simulink model "dsa2k_iwave_rfi"  (R2021a)
settings: Solver=VariableStepAuto  StartTime=0.0  StopTime=10.0  RelTol=1e-3
undefined symbols (not defined in the file): datetime, i, posixtime
libraries: xbsIndex_r4 x3053, casper_library_misc x61, rtr_casper_dsp_lib x31, xps_library x1
(part 5 of 43)

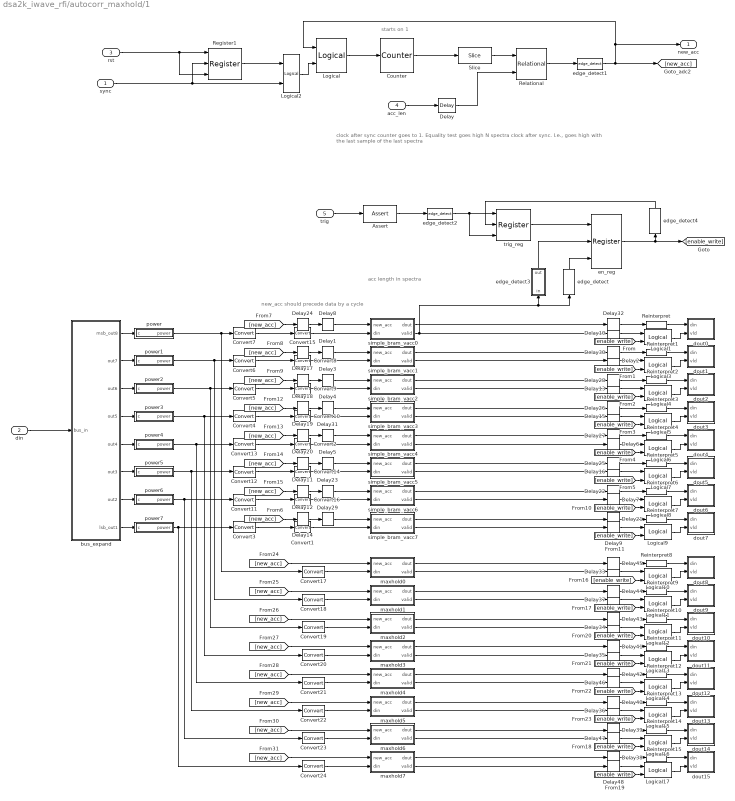
== system dsa2k_iwave_rfi/autocorr_maxhold/1 ==
  note: new_acc should precede data by a cycle
  note: acc length in spectra
  note: clock after sync counter goes to 1.
      |
      | Equality test goes high N spectra clock after sync. I.e., goes high with the last sample of the last spectra
  note: starts on 1
  sync : Inport
  din : Inport  Port=2
  rst : Inport  Port=3
  acc_len : Inport  Port=4
  trig : Inport  Port=5
  Assert : xbsIndex_r4/Assert  assert_type=off  type_source=Explicitly  gui_display_data_type=Fixed-point  arith_type="Signed  (2's comp)"  n_bits=16  bin_pt=14  preci_type=Single  exp_width=8  frac_width=24  assert_rate=on  rate_source=Explicitly  period=1  output_port=on  block_type=assert
  Convert{1..2,8..10,14..16} (8 alike) : xbsIndex_r4/Convert  gui_display_data_type=Floating-point  arith_type=Floating-point  n_bits=31  bin_pt=28  float_type=Single  exp_bits=8  fraction_bits=24  quantization="Round  (unbiased: Even Values)"  overflow=Wrap  en=off  latency=3  pipeline=on  dbl_ovrd=off  block_type=convert
  Convert{3..7,11..13} (8 alike) : xbsIndex_r4/Convert  gui_display_data_type=Fixed-point  arith_type="Signed  (2's comp)"  n_bits=37  bin_pt=34  float_type=Single  exp_bits=8  fraction_bits=24  quantization=Truncate  overflow=Wrap  en=off  latency=0  pipeline=off  dbl_ovrd=off  block_type=convert
  Convert{17..24} (8 alike) : xbsIndex_r4/Convert  gui_display_data_type=Fixed-point  arith_type=Unsigned  n_bits=32  bin_pt=30  float_type=Single  exp_bits=8  fraction_bits=24  quantization=Truncate  overflow=Wrap  en=off  latency=0  pipeline=off  dbl_ovrd=off  block_type=convert
  Counter : xbsIndex_r4/Counter  cnt_type=Free Running  cnt_to=Inf  operation=Up  start_count=1  cnt_by_val=1  arith_type=Unsigned  n_bits=30  bin_pt=0  load_pin=off  rst=on  en=off  explicit_period=on  period=1  use_behavioral_HDL=off  implementation=Fabric  dbl_ovrd=off  block_type=counter
  Delay{,2,6..7,9..10,13,15..16,33..37,46..48} (17 alike) : xbsIndex_r4/Delay  rst=off  infoeditControl=Selection of Reset will increase slice count due to use of real FFs and instead of SRLs  en=off  latency=1  reg_retiming=off  dbl_ovrd=off  block_type=delay
  Delay{1,3..5,8,23,29,31} (8 alike) : xbsIndex_r4/Delay  rst=off  infoeditControl=Selection of Reset will increase slice count due to use of real FFs and instead of SRLs  en=off  latency=4  reg_retiming=on  dbl_ovrd=off  block_type=delay
  Delay{11..12,14,17..20,24} (8 alike) : xbsIndex_r4/Delay  rst=off  infoeditControl=Selection of Reset will increase slice count due to use of real FFs and instead of SRLs  en=off  latency=3  reg_retiming=on  dbl_ovrd=off  block_type=delay
  Delay{21..22,25..28,30,32,38..45} (16 alike) : xbsIndex_r4/Delay  rst=off  infoeditControl=Selection of Reset will increase slice count due to use of real FFs and instead of SRLs  en=off  latency=1  reg_retiming=on  dbl_ovrd=off  block_type=delay
  Logical : xbsIndex_r4/Logical  logical_function=OR  inputs=2  en=off  latency=0  precision=Full  arith_type=Unsigned  n_bits=16  bin_pt=0  align_bp=on  dbl_ovrd=off  block_type=logical
  Logical{1..17} (17 alike) : xbsIndex_r4/Logical  logical_function=AND  inputs=2  en=off  latency=0  precision=Full  arith_type=Unsigned  n_bits=16  bin_pt=0  align_bp=on  dbl_ovrd=off  block_type=logical
  Register1 : xbsIndex_r4/Register  init=0  rst=on  en=on  dbl_ovrd=off  block_type=register
  Reinterpret{,1..15} (16 alike) : xbsIndex_r4/Reinterpret  force_arith_type=on  arith_type=Unsigned  force_bin_pt=on  bin_pt=0  block_type=reinterpret
  Relational : xbsIndex_r4/Relational  mode=a=b  op_type=Bool  en=off  latency=0  dbl_ovrd=off  block_type=relational
  Slice : xbsIndex_r4/Slice  nbits=30-nchan_bits-npol_bits  boolean_output=off  mode=Lower Bit Location + Width  bit1=0  base1=MSB of Input  bit0=nchan_bits + npol_bits  base0=LSB of Input  dbl_ovrd=off  block_type=slice
  bus_expand : Subsystem  AncestorBlock=casper_library_flow_control/bus_expand  mask(bus_expand){mode=divisions of equal size, outputNum=8, outputWidth=36, outputBinaryPt=0, outputArithmeticType=0, show_format=off, outputToWorkspace=off, variablePrefix=out, outputToModelAsWell=on}
      mask prompts: outputNum "Number of outputs:"; outputWidth "Output width:"; outputBinaryPt "Output binary point position:"; outputArithmeticType "Output arithmetic type (ufix=0, fix=1, bool=2):"; show_format "Print format string?"; outputToWorkspace "Output to workspace?"; variablePrefix "Variable name prefix:"; outputToModelAsWell "Output to model as well?"
      mask help:
      | Expands a 'bus' made using a bus_create or Xilinx
      | concat block.
      | The input will be divided into the specified number
      | of outputs with the specified arithmetic types.
      | Divisions are made from most significant bit.
      mask init: same as dsa2k_iwave_rfi/autocorr_maxhold/bus_expand
      settings: AttributesFormatString=8 outputs
      mask TypeOptions mode: divisions of equal size | divisions of arbitrary size
      mask Callback mode: %bus_expand_callback();
      mask Callback outputWidth: %bus_expand_callback();
      mask Callback outputToWorkspace: %bus_expand_callback();
  dout0 : Subsystem
  dout1 : Subsystem
  dout10 : Subsystem
  dout11 : Subsystem
  dout12 : Subsystem
  dout13 : Subsystem
  dout14 : Subsystem
  dout15 : Subsystem
  dout2 : Subsystem
  dout3 : Subsystem
  dout4 : Subsystem
  dout5 : Subsystem
  dout6 : Subsystem
  dout7 : Subsystem
  dout8 : Subsystem
  dout9 : Subsystem
  edge_detect{,1..2,4} (4 alike) : casper_library_misc/edge_detect  edge=Rising  polarity=Active High  x_in=[0 0.08 0.08 0.16 0.16 0.24 0.24 0.32 0.32 0.4]  y_in="[-1 -1  1  1  1  1  1  1  1  1]"  x_out=[0.6 0.68 0.68 0.76 0.76 0.84 0.84 0.92 0.92 1]  y_out="[-1 -1  1  1 -1 -1 -1 -1 -1 -1]"
  edge_detect3 : Subsystem  AncestorBlock=casper_library_misc/edge_detect  mask(edge_detect){edge=Falling, polarity=Active High, x_in=[0 0.08 0.08 0.16 0.16 0.24 0.24 0.32 0.32 0.4], y_in=[-1 -1  1  1  1  1  1  1  1  1], x_out=[0.6 0.68 0.68 0.76 0.76 0.84 0.84 0.92 0.92 1], y_out=[-1 -1  1  1 -1 -1 -1 -1 -1 -1]}
      mask prompts: edge "Edge Type"; polarity "Output Polarity"; x_in "Input X Positions"; y_in "Input Y Positions"; x_out "Output X Positions"; y_out "Output Y Positions"
      mask help: Output is active for one-cycle after each edge of the specified type (i.e. rising, falling or both).
      mask init: same as dsa2k_iwave_rfi/sync/ed1
      settings: AttributesFormatString=|
      | falling edges
      | active high
      mask Help: Output is active for one-cycle after each edge of the specified type (i.e. rising, falling, or both).  Latency is zero.
      mask TypeOptions edge: Rising | Falling | Both
      mask TypeOptions polarity: Active High | Active Low
      mask Display:
      | plot(x_in_num,0.5+y_in_num*0.2);
      | plot(x_out_num,0.5+y_out_num*0.2);
  en_reg : xbsIndex_r4/Register  init=0  rst=on  en=on  dbl_ovrd=off  block_type=register
  maxhold0 : Subsystem  AncestorBlock=casper_library_accumulators/simple_bram_vacc  mask(simple_bram_vacc){vec_len=2^(nchan_bits + npol_bits), arith_type=Unsigned, n_bits=32, bin_pt=30}
      mask prompts: vec_len "Vector length:"; arith_type "Output type:"; n_bits "Bit width (output):"; bin_pt "Binary point (output):"
      mask help: This simple vector accumulator is based on a shift register. It outputs its previous accumulated vector after a new_acc pulse is received.
      mask init:
      | % simple_bram_vacc_init(gcb, ...
      | %     'vec_len', vec_len, ...
      | %     'arith_type', arith_type, ...
      | %     'n_bits', n_bits, ...
      | %     'bin_pt', bin_pt);
      mask TypeOptions arith_type: Signed | Unsigned
  maxhold1 : Subsystem  AncestorBlock=casper_library_accumulators/simple_bram_vacc  mask(simple_bram_vacc){vec_len=2^(nchan_bits + npol_bits), arith_type=Unsigned, n_bits=32, bin_pt=30}
      mask prompts: vec_len "Vector length:"; arith_type "Output type:"; n_bits "Bit width (output):"; bin_pt "Binary point (output):"
      mask help: This simple vector accumulator is based on a shift register. It outputs its previous accumulated vector after a new_acc pulse is received.
      mask init:
      | % simple_bram_vacc_init(gcb, ...
      | %     'vec_len', vec_len, ...
      | %     'arith_type', arith_type, ...
      | %     'n_bits', n_bits, ...
      | %     'bin_pt', bin_pt);
      mask TypeOptions arith_type: Signed | Unsigned
  maxhold2 : Subsystem  AncestorBlock=casper_library_accumulators/simple_bram_vacc  mask(simple_bram_vacc){vec_len=2^(nchan_bits + npol_bits), arith_type=Unsigned, n_bits=32, bin_pt=30}
      mask prompts: vec_len "Vector length:"; arith_type "Output type:"; n_bits "Bit width (output):"; bin_pt "Binary point (output):"
      mask help: This simple vector accumulator is based on a shift register. It outputs its previous accumulated vector after a new_acc pulse is received.
      mask init:
      | % simple_bram_vacc_init(gcb, ...
      | %     'vec_len', vec_len, ...
      | %     'arith_type', arith_type, ...
      | %     'n_bits', n_bits, ...
      | %     'bin_pt', bin_pt);
      mask TypeOptions arith_type: Signed | Unsigned
  maxhold3 : Subsystem  AncestorBlock=casper_library_accumulators/simple_bram_vacc  mask(simple_bram_vacc){vec_len=2^(nchan_bits + npol_bits), arith_type=Unsigned, n_bits=32, bin_pt=30}
      mask prompts: vec_len "Vector length:"; arith_type "Output type:"; n_bits "Bit width (output):"; bin_pt "Binary point (output):"
      mask help: This simple vector accumulator is based on a shift register. It outputs its previous accumulated vector after a new_acc pulse is received.
      mask init:
      | % simple_bram_vacc_init(gcb, ...
      | %     'vec_len', vec_len, ...
      | %     'arith_type', arith_type, ...
      | %     'n_bits', n_bits, ...
      | %     'bin_pt', bin_pt);
      mask TypeOptions arith_type: Signed | Unsigned
  maxhold4 : Subsystem  AncestorBlock=casper_library_accumulators/simple_bram_vacc  mask(simple_bram_vacc){vec_len=2^(nchan_bits + npol_bits), arith_type=Unsigned, n_bits=32, bin_pt=30}
      mask prompts: vec_len "Vector length:"; arith_type "Output type:"; n_bits "Bit width (output):"; bin_pt "Binary point (output):"
      mask help: This simple vector accumulator is based on a shift register. It outputs its previous accumulated vector after a new_acc pulse is received.
      mask init:
      | % simple_bram_vacc_init(gcb, ...
      | %     'vec_len', vec_len, ...
      | %     'arith_type', arith_type, ...
      | %     'n_bits', n_bits, ...
      | %     'bin_pt', bin_pt);
      mask TypeOptions arith_type: Signed | Unsigned
  maxhold5 : Subsystem  AncestorBlock=casper_library_accumulators/simple_bram_vacc  mask(simple_bram_vacc){vec_len=2^(nchan_bits + npol_bits), arith_type=Unsigned, n_bits=32, bin_pt=30}
      mask prompts: vec_len "Vector length:"; arith_type "Output type:"; n_bits "Bit width (output):"; bin_pt "Binary point (output):"
      mask help: This simple vector accumulator is based on a shift register. It outputs its previous accumulated vector after a new_acc pulse is received.
      mask init:
      | % simple_bram_vacc_init(gcb, ...
      | %     'vec_len', vec_len, ...
      | %     'arith_type', arith_type, ...
      | %     'n_bits', n_bits, ...
      | %     'bin_pt', bin_pt);
      mask TypeOptions arith_type: Signed | Unsigned
  maxhold6 : Subsystem  AncestorBlock=casper_library_accumulators/simple_bram_vacc  mask(simple_bram_vacc){vec_len=2^(nchan_bits + npol_bits), arith_type=Unsigned, n_bits=32, bin_pt=30}
      mask prompts: vec_len "Vector length:"; arith_type "Output type:"; n_bits "Bit width (output):"; bin_pt "Binary point (output):"
      mask help: This simple vector accumulator is based on a shift register. It outputs its previous accumulated vector after a new_acc pulse is received.
      mask init:
      | % simple_bram_vacc_init(gcb, ...
      | %     'vec_len', vec_len, ...
      | %     'arith_type', arith_type, ...
      | %     'n_bits', n_bits, ...
      | %     'bin_pt', bin_pt);
      mask TypeOptions arith_type: Signed | Unsigned
  maxhold7 : Subsystem  AncestorBlock=casper_library_accumulators/simple_bram_vacc  mask(simple_bram_vacc){vec_len=2^(nchan_bits + npol_bits), arith_type=Unsigned, n_bits=32, bin_pt=30}
      mask prompts: vec_len "Vector length:"; arith_type "Output type:"; n_bits "Bit width (output):"; bin_pt "Binary point (output):"
      mask help: This simple vector accumulator is based on a shift register. It outputs its previous accumulated vector after a new_acc pulse is received.
      mask init:
      | % simple_bram_vacc_init(gcb, ...
      | %     'vec_len', vec_len, ...
      | %     'arith_type', arith_type, ...
      | %     'n_bits', n_bits, ...
      | %     'bin_pt', bin_pt);
      mask TypeOptions arith_type: Signed | Unsigned
  power : Subsystem  mask(power){BitWidth=18, add_latency=1, mult_latency=3}
      mask prompts: BitWidth "Bit Width"; add_latency "Add Latency"; mult_latency "Mult Latency"
      mask help: Squares real and imaginary components of complex input and adds them.
      mask Help: eval('xlWeb(''http://casper.berkeley.edu/wiki/Power'')')
      mask Display:
      | port_label('input', 1, 'c');
      | port_label('output', 1, 'power');
      | disp(['Z^-', num2str(mult_latency+add_latency)]);
  power1 : Subsystem  mask(power){BitWidth=18, add_latency=1, mult_latency=3}
      mask prompts: BitWidth "Bit Width"; add_latency "Add Latency"; mult_latency "Mult Latency"
      mask help: Squares real and imaginary components of complex input and adds them.
      mask Help: eval('xlWeb(''http://casper.berkeley.edu/wiki/Power'')')
      mask Display:
      | port_label('input', 1, 'c');
      | port_label('output', 1, 'power');
      | disp(['Z^-', num2str(mult_latency+add_latency)]);
  power2 : Subsystem  mask(power){BitWidth=18, add_latency=1, mult_latency=3}
      mask prompts: BitWidth "Bit Width"; add_latency "Add Latency"; mult_latency "Mult Latency"
      mask help: Squares real and imaginary components of complex input and adds them.
      mask Help: eval('xlWeb(''http://casper.berkeley.edu/wiki/Power'')')
      mask Display:
      | port_label('input', 1, 'c');
      | port_label('output', 1, 'power');
      | disp(['Z^-', num2str(mult_latency+add_latency)]);
  power3 : Subsystem  mask(power){BitWidth=18, add_latency=1, mult_latency=3}
      mask prompts: BitWidth "Bit Width"; add_latency "Add Latency"; mult_latency "Mult Latency"
      mask help: Squares real and imaginary components of complex input and adds them.
      mask Help: eval('xlWeb(''http://casper.berkeley.edu/wiki/Power'')')
      mask Display:
      | port_label('input', 1, 'c');
      | port_label('output', 1, 'power');
      | disp(['Z^-', num2str(mult_latency+add_latency)]);
  power4 : Subsystem  mask(power){BitWidth=18, add_latency=1, mult_latency=3}
      mask prompts: BitWidth "Bit Width"; add_latency "Add Latency"; mult_latency "Mult Latency"
      mask help: Squares real and imaginary components of complex input and adds them.
      mask Help: eval('xlWeb(''http://casper.berkeley.edu/wiki/Power'')')
      mask Display:
      | port_label('input', 1, 'c');
      | port_label('output', 1, 'power');
      | disp(['Z^-', num2str(mult_latency+add_latency)]);
  power5 : Subsystem  mask(power){BitWidth=18, add_latency=1, mult_latency=3}
      mask prompts: BitWidth "Bit Width"; add_latency "Add Latency"; mult_latency "Mult Latency"
      mask help: Squares real and imaginary components of complex input and adds them.
      mask Help: eval('xlWeb(''http://casper.berkeley.edu/wiki/Power'')')
      mask Display:
      | port_label('input', 1, 'c');
      | port_label('output', 1, 'power');
      | disp(['Z^-', num2str(mult_latency+add_latency)]);
  power6 : Subsystem  mask(power){BitWidth=18, add_latency=1, mult_latency=3}
      mask prompts: BitWidth "Bit Width"; add_latency "Add Latency"; mult_latency "Mult Latency"
      mask help: Squares real and imaginary components of complex input and adds them.
      mask Help: eval('xlWeb(''http://casper.berkeley.edu/wiki/Power'')')
      mask Display:
      | port_label('input', 1, 'c');
      | port_label('output', 1, 'power');
      | disp(['Z^-', num2str(mult_latency+add_latency)]);
  power7 : Subsystem  mask(power){BitWidth=18, add_latency=1, mult_latency=3}
      mask prompts: BitWidth "Bit Width"; add_latency "Add Latency"; mult_latency "Mult Latency"
      mask help: Squares real and imaginary components of complex input and adds them.
      mask Help: eval('xlWeb(''http://casper.berkeley.edu/wiki/Power'')')
      mask Display:
      | port_label('input', 1, 'c');
      | port_label('output', 1, 'power');
      | disp(['Z^-', num2str(mult_latency+add_latency)]);
  simple_bram_vacc0 : Subsystem  AncestorBlock=casper_library_accumulators/simple_bram_vacc  mask(simple_bram_vacc){vec_len=2^(nchan_bits + npol_bits), arith_type=Signed, n_bits=30 + 17, bin_pt=28}
      mask prompts: vec_len "Vector length:"; arith_type "Output type:"; n_bits "Bit width (output):"; bin_pt "Binary point (output):"
      mask help: This simple vector accumulator is based on a shift register. It outputs its previous accumulated vector after a new_acc pulse is received.
      mask init:
      | simple_bram_vacc_init(gcb, ...
      |     'vec_len', vec_len, ...
      |     'arith_type', arith_type, ...
      |     'n_bits', n_bits, ...
      |     'bin_pt', bin_pt);
      mask TypeOptions arith_type: Signed | Unsigned
  simple_bram_vacc1 : Subsystem  AncestorBlock=casper_library_accumulators/simple_bram_vacc  mask(simple_bram_vacc){vec_len=2^(nchan_bits + npol_bits), arith_type=Signed, n_bits=30 + 17, bin_pt=28}
      mask prompts: vec_len "Vector length:"; arith_type "Output type:"; n_bits "Bit width (output):"; bin_pt "Binary point (output):"
      mask help: This simple vector accumulator is based on a shift register. It outputs its previous accumulated vector after a new_acc pulse is received.
      mask init:
      | simple_bram_vacc_init(gcb, ...
      |     'vec_len', vec_len, ...
      |     'arith_type', arith_type, ...
      |     'n_bits', n_bits, ...
      |     'bin_pt', bin_pt);
      mask TypeOptions arith_type: Signed | Unsigned
  simple_bram_vacc2 : Subsystem  AncestorBlock=casper_library_accumulators/simple_bram_vacc  mask(simple_bram_vacc){vec_len=2^(nchan_bits + npol_bits), arith_type=Signed, n_bits=30 + 17, bin_pt=28}
      mask prompts: vec_len "Vector length:"; arith_type "Output type:"; n_bits "Bit width (output):"; bin_pt "Binary point (output):"
      mask help: This simple vector accumulator is based on a shift register. It outputs its previous accumulated vector after a new_acc pulse is received.
      mask init:
      | simple_bram_vacc_init(gcb, ...
      |     'vec_len', vec_len, ...
      |     'arith_type', arith_type, ...
      |     'n_bits', n_bits, ...
      |     'bin_pt', bin_pt);
      mask TypeOptions arith_type: Signed | Unsigned
  simple_bram_vacc3 : Subsystem  AncestorBlock=casper_library_accumulators/simple_bram_vacc  mask(simple_bram_vacc){vec_len=2^(nchan_bits + npol_bits), arith_type=Signed, n_bits=30 + 17, bin_pt=28}
      mask prompts: vec_len "Vector length:"; arith_type "Output type:"; n_bits "Bit width (output):"; bin_pt "Binary point (output):"
      mask help: This simple vector accumulator is based on a shift register. It outputs its previous accumulated vector after a new_acc pulse is received.
      mask init:
      | simple_bram_vacc_init(gcb, ...
      |     'vec_len', vec_len, ...
      |     'arith_type', arith_type, ...
      |     'n_bits', n_bits, ...
      |     'bin_pt', bin_pt);
      mask TypeOptions arith_type: Signed | Unsigned
  simple_bram_vacc4 : Subsystem  AncestorBlock=casper_library_accumulators/simple_bram_vacc  mask(simple_bram_vacc){vec_len=2^(nchan_bits + npol_bits), arith_type=Signed, n_bits=30 + 17, bin_pt=28}
      mask prompts: vec_len "Vector length:"; arith_type "Output type:"; n_bits "Bit width (output):"; bin_pt "Binary point (output):"
      mask help: This simple vector accumulator is based on a shift register. It outputs its previous accumulated vector after a new_acc pulse is received.
      mask init:
      | simple_bram_vacc_init(gcb, ...
      |     'vec_len', vec_len, ...
      |     'arith_type', arith_type, ...
      |     'n_bits', n_bits, ...
      |     'bin_pt', bin_pt);
      mask TypeOptions arith_type: Signed | Unsigned
  simple_bram_vacc5 : Subsystem  AncestorBlock=casper_library_accumulators/simple_bram_vacc  mask(simple_bram_vacc){vec_len=2^(nchan_bits + npol_bits), arith_type=Signed, n_bits=30 + 17, bin_pt=28}
      mask prompts: vec_len "Vector length:"; arith_type "Output type:"; n_bits "Bit width (output):"; bin_pt "Binary point (output):"
      mask help: This simple vector accumulator is based on a shift register. It outputs its previous accumulated vector after a new_acc pulse is received.
      mask init:
      | simple_bram_vacc_init(gcb, ...
      |     'vec_len', vec_len, ...
      |     'arith_type', arith_type, ...
      |     'n_bits', n_bits, ...
      |     'bin_pt', bin_pt);
      mask TypeOptions arith_type: Signed | Unsigned
  simple_bram_vacc6 : Subsystem  AncestorBlock=casper_library_accumulators/simple_bram_vacc  mask(simple_bram_vacc){vec_len=2^(nchan_bits + npol_bits), arith_type=Signed, n_bits=30 + 17, bin_pt=28}
      mask prompts: vec_len "Vector length:"; arith_type "Output type:"; n_bits "Bit width (output):"; bin_pt "Binary point (output):"
      mask help: This simple vector accumulator is based on a shift register. It outputs its previous accumulated vector after a new_acc pulse is received.
      mask init:
      | simple_bram_vacc_init(gcb, ...
      |     'vec_len', vec_len, ...
      |     'arith_type', arith_type, ...
      |     'n_bits', n_bits, ...
      |     'bin_pt', bin_pt);
      mask TypeOptions arith_type: Signed | Unsigned
  simple_bram_vacc7 : Subsystem  AncestorBlock=casper_library_accumulators/simple_bram_vacc  mask(simple_bram_vacc){vec_len=2^(nchan_bits + npol_bits), arith_type=Signed, n_bits=30 + 17, bin_pt=28}
      mask prompts: vec_len "Vector length:"; arith_type "Output type:"; n_bits "Bit width (output):"; bin_pt "Binary point (output):"
      mask help: This simple vector accumulator is based on a shift register. It outputs its previous accumulated vector after a new_acc pulse is received.
      mask init:
      | simple_bram_vacc_init(gcb, ...
      |     'vec_len', vec_len, ...
      |     'arith_type', arith_type, ...
      |     'n_bits', n_bits, ...
      |     'bin_pt', bin_pt);
      mask TypeOptions arith_type: Signed | Unsigned
  trig_reg : xbsIndex_r4/Register  init=0  rst=on  en=on  dbl_ovrd=off  block_type=register
  new_acc : Outport  VectorParamsAs1DForOutWhenUnconnected=off
  wires:
  Delay31/1 -> simple_bram_vacc4/1(new_acc)
  Delay5/1 -> simple_bram_vacc5/1(new_acc)
  Delay23/1 -> simple_bram_vacc6/1(new_acc)
  Delay29/1 -> simple_bram_vacc7/1(new_acc)
  power7/1(power) -> Convert3/1, Convert24/1
  power6/1(power) -> Convert11/1, Convert23/1
  power5/1(power) -> Convert12/1, Convert22/1
  power4/1(power) -> Convert13/1, Convert21/1
  [new_acc] -> Delay14/1
  [new_acc] -> Delay12/1
  [new_acc] -> Delay11/1
  [new_acc] -> Delay20/1
  Logical6/1 -> dout4/2(vld)
  [enable_write] -> Logical6/2
  [enable_write] -> Logical7/2
  Logical7/1 -> dout5/2(vld)
  Logical8/1 -> dout6/2(vld)
  [enable_write] -> Logical8/2
  [enable_write] -> Logical9/2
  Logical9/1 -> dout7/2(vld)
  simple_bram_vacc4/1(dout) -> Delay27/1
  simple_bram_vacc5/1(dout) -> Delay25/1
  simple_bram_vacc6/1(dout) -> Delay22/1
  simple_bram_vacc6/2(valid) -> Delay7/1
  simple_bram_vacc7/1(dout) -> Delay21/1
  simple_bram_vacc7/2(valid) -> Delay9/1
  simple_bram_vacc5/2(valid) -> Delay16/1
  simple_bram_vacc4/2(valid) -> Delay6/1
  Delay14/1 -> Delay29/1
  Convert1/1 -> simple_bram_vacc7/2(din)
  Delay12/1 -> Delay23/1
  Convert16/1 -> simple_bram_vacc6/2(din)
  Convert14/1 -> simple_bram_vacc5/2(din)
  Delay11/1 -> Delay5/1
  Delay20/1 -> Delay31/1
  Convert2/1 -> simple_bram_vacc4/2(din)
  Delay27/1 -> Reinterpret4/1
  Delay6/1 -> Logical6/1
  Delay25/1 -> Reinterpret5/1
  Delay16/1 -> Logical7/1
  Delay22/1 -> Reinterpret6/1
  Delay7/1 -> Logical8/1
  Delay9/1 -> Logical9/1
  Delay21/1 -> Reinterpret7/1
  Convert3/1 -> Convert1/1
  Convert11/1 -> Convert16/1
  Convert12/1 -> Convert14/1
  Convert13/1 -> Convert2/1
  Reinterpret4/1 -> dout4/1(din)
  Reinterpret5/1 -> dout5/1(din)
  Reinterpret6/1 -> dout6/1(din)
  Reinterpret7/1 -> dout7/1(din)
  Reinterpret3/1 -> dout3/1(din)
  Reinterpret2/1 -> dout2/1(din)
  Reinterpret1/1 -> dout1/1(din)
  Reinterpret/1 -> dout0/1(din)
  Convert7/1 -> Convert15/1
  Convert6/1 -> Convert8/1
  Convert5/1 -> Convert9/1
  Convert4/1 -> Convert10/1
  Delay26/1 -> Reinterpret3/1
  Delay15/1 -> Logical5/1
  Delay13/1 -> Logical4/1
  Delay28/1 -> Reinterpret2/1
  Delay2/1 -> Logical3/1
  Delay30/1 -> Reinterpret1/1
  Delay10/1 -> Logical1/1
  Delay32/1 -> Reinterpret/1
  Convert15/1 -> simple_bram_vacc0/2(din)
  Delay24/1 -> Delay8/1
  Delay17/1 -> Delay1/1
  Convert8/1 -> simple_bram_vacc1/2(din)
  Convert9/1 -> simple_bram_vacc2/2(din)
  Delay18/1 -> Delay3/1
  Convert10/1 -> simple_bram_vacc3/2(din)
  Delay19/1 -> Delay4/1
  simple_bram_vacc0/2(valid) -> edge_detect3/1(in), edge_detect/1, Delay10/1
  simple_bram_vacc1/2(valid) -> Delay2/1
  simple_bram_vacc3/2(valid) -> Delay15/1
  simple_bram_vacc3/1(dout) -> Delay26/1
  simple_bram_vacc2/2(valid) -> Delay13/1
  simple_bram_vacc2/1(dout) -> Delay28/1
  simple_bram_vacc1/1(dout) -> Delay30/1
  simple_bram_vacc0/1(dout) -> Delay32/1
  Assert/1 -> edge_detect2/1
  trig/1 -> Assert/1
  Logical5/1 -> dout3/2(vld)
  [enable_write] -> Logical5/2
  [enable_write] -> Logical4/2
  Logical4/1 -> dout2/2(vld)
  Logical3/1 -> dout1/2(vld)
  [enable_write] -> Logical3/2
  [enable_write] -> Logical1/2
  en_reg/1 -> edge_detect4/1, [enable_write]
  Logical1/1 -> dout0/2(vld)
  edge_detect4/1 -> trig_reg/2
  edge_detect3/1(out) -> en_reg/2
  edge_detect/1 -> en_reg/3
  edge_detect2/1 -> trig_reg/1, trig_reg/3
  trig_reg/1 -> en_reg/1
  sync/1 -> Register1/2, Logical2/2
  Register1/1 -> Logical2/1
  rst/1 -> Register1/3, Register1/1
  edge_detect1/1 -> Logical/1, new_acc/1, [new_acc]
  Logical/1 -> Counter/1
  Counter/1 -> Slice/1
  [new_acc] -> Delay24/1
  [new_acc] -> Delay17/1
  [new_acc] -> Delay18/1
  [new_acc] -> Delay19/1
  power/1(power) -> Convert17/1, Convert7/1
  power1/1(power) -> Convert6/1, Convert18/1
  power2/1(power) -> Convert5/1, Convert19/1
  power3/1(power) -> Convert4/1, Convert20/1
  din/1 -> bus_expand/1(bus_in)
  Slice/1 -> Relational/1
  Relational/1 -> edge_detect1/1
  Logical2/1 -> Logical/2
  acc_len/1 -> Delay/1
  Delay4/1 -> simple_bram_vacc3/1(new_acc)
  Delay3/1 -> simple_bram_vacc2/1(new_acc)
  Delay1/1 -> simple_bram_vacc1/1(new_acc)
  Delay8/1 -> simple_bram_vacc0/1(new_acc)
  Delay/1 -> Relational/2
  bus_expand/1(msb_out8) -> power/1(c)
  bus_expand/2(out7) -> power1/1(c)
  bus_expand/3(out6) -> power2/1(c)
  bus_expand/4(out5) -> power3/1(c)
  bus_expand/5(out4) -> power4/1(c)
  bus_expand/6(out3) -> power5/1(c)
  bus_expand/7(out2) -> power6/1(c)
  bus_expand/8(lsb_out1) -> power7/1(c)
  Logical10/1 -> dout8/2(vld)
  [enable_write] -> Logical10/2
  [enable_write] -> Logical11/2
  Logical11/1 -> dout9/2(vld)
  Logical12/1 -> dout10/2(vld)
  [enable_write] -> Logical12/2
  [enable_write] -> Logical13/2
  Logical13/1 -> dout11/2(vld)
  maxhold0/1(dout) -> Delay45/1
  maxhold1/1(dout) -> Delay44/1
  maxhold2/1(dout) -> Delay43/1
  maxhold2/2(valid) -> Delay34/1
  maxhold3/1(dout) -> Delay41/1
  maxhold3/2(valid) -> Delay35/1
  maxhold1/2(valid) -> Delay37/1
  maxhold0/2(valid) -> Delay33/1
  Delay45/1 -> Reinterpret8/1
  Delay33/1 -> Logical10/1
  Delay44/1 -> Reinterpret9/1
  Delay37/1 -> Logical11/1
  Delay43/1 -> Reinterpret10/1
  Delay34/1 -> Logical12/1
  Delay35/1 -> Logical13/1
  Delay41/1 -> Reinterpret11/1
  Reinterpret8/1 -> dout8/1(din)
  Reinterpret9/1 -> dout9/1(din)
  Reinterpret10/1 -> dout10/1(din)
  Reinterpret11/1 -> dout11/1(din)
  Reinterpret15/1 -> dout15/1(din)
  Reinterpret14/1 -> dout14/1(din)
  Reinterpret13/1 -> dout13/1(din)
  Reinterpret12/1 -> dout12/1(din)
  Delay38/1 -> Reinterpret15/1
  Delay48/1 -> Logical17/1
  Delay47/1 -> Logical16/1
  Delay39/1 -> Reinterpret14/1
  Delay36/1 -> Logical15/1
  Delay40/1 -> Reinterpret13/1
  Delay46/1 -> Logical14/1
  Delay42/1 -> Reinterpret12/1
  maxhold4/2(valid) -> Delay46/1
  maxhold5/2(valid) -> Delay36/1
  maxhold7/2(valid) -> Delay48/1
  maxhold7/1(dout) -> Delay38/1
  maxhold6/2(valid) -> Delay47/1
  maxhold6/1(dout) -> Delay39/1
  maxhold5/1(dout) -> Delay40/1
  maxhold4/1(dout) -> Delay42/1
  Logical17/1 -> dout15/2(vld)
  [enable_write] -> Logical17/2
  [enable_write] -> Logical16/2
  Logical16/1 -> dout14/2(vld)
  Logical15/1 -> dout13/2(vld)
  [enable_write] -> Logical15/2
  [enable_write] -> Logical14/2
  Logical14/1 -> dout12/2(vld)
  [new_acc] -> maxhold0/1(new_acc)
  Convert17/1 -> maxhold0/2(din)
  [new_acc] -> maxhold1/1(new_acc)
  Convert18/1 -> maxhold1/2(din)
  [new_acc] -> maxhold2/1(new_acc)
  Convert19/1 -> maxhold2/2(din)
  [new_acc] -> maxhold3/1(new_acc)
  Convert20/1 -> maxhold3/2(din)
  Convert21/1 -> maxhold4/2(din)
  [new_acc] -> maxhold4/1(new_acc)
  [new_acc] -> maxhold5/1(new_acc)
  Convert22/1 -> maxhold5/2(din)
  Convert23/1 -> maxhold6/2(din)
  [new_acc] -> maxhold6/1(new_acc)
  [new_acc] -> maxhold7/1(new_acc)
  Convert24/1 -> maxhold7/2(din)

== system dsa2k_iwave_rfi/autocorr_maxhold/acc_cnt ==
  out_reg : Inport
  assert_reg : xbsIndex_r4/Assert  assert_type=on  type_source=Explicitly  gui_display_data_type=Fixed-point  arith_type=Unsigned  n_bits=32  bin_pt=0  preci_type=Single  exp_width=8  frac_width=24  assert_rate=off  rate_source=Explicitly  period=1  output_port=on  block_type=assert
  cast_gw : xbsIndex_r4/Convert  gui_display_data_type=Fixed-point  arith_type=Unsigned  n_bits=32  bin_pt=0  float_type=Single  exp_bits=8  fraction_bits=24  quantization=Truncate  overflow=Wrap  en=off  latency=1  pipeline=off  dbl_ovrd=off  block_type=convert
  dsa2k_iwave_rfi_autocorr_maxhold_acc_cnt_user_data_in : xbsIndex_r4/Gateway Out  inherit_from_input=off  hdl_port=on  rows=1  columns=1  UseAsDAC=off  DACChannel='1'  interface=None  automatic_assignment=on  address_offset=hex2dec('00')  intf_name=''  intf_description=''  timing_constraint=None  locs_specified=off  LOCs={}  io_standard={}  block_type=gatewayout
  io_delay : xbsIndex_r4/Delay  rst=off  infoeditControl=Selection of Reset will increase slice count due to use of real FFs and instead of SRLs  en=off  latency=0  reg_retiming=on  dbl_ovrd=off  block_type=delay
  reint1 : xbsIndex_r4/Reinterpret  force_arith_type=on  arith_type=Unsigned  force_bin_pt=on  bin_pt=0  block_type=reinterpret
  sim_out : Terminator
  sim_out_reg_gw : xbsIndex_r4/Gateway Out  inherit_from_input=off  hdl_port=off  rows=1  columns=1  UseAsDAC=off  DACChannel='1'  interface=None  automatic_assignment=on  address_offset=hex2dec('00')  intf_name=''  intf_description=''  timing_constraint=None  locs_specified=off  LOCs={}  io_standard={}  block_type=gatewayout
  sim_out_reg_sim_delay : xbsIndex_r4/Delay  rst=off  infoeditControl=Selection of Reset will increase slice count due to use of real FFs and instead of SRLs  en=off  latency=1  reg_retiming=on  dbl_ovrd=off  block_type=delay
  sim_out_reg : Outport  VectorParamsAs1DForOutWhenUnconnected=off
  wires:
  sim_out_reg_sim_delay/1 -> sim_out_reg_gw/1
  sim_out_reg_gw/1 -> sim_out_reg/1
  io_delay/1 -> cast_gw/1
  cast_gw/1 -> dsa2k_iwave_rfi_autocorr_maxhold_acc_cnt_user_data_in/1
  dsa2k_iwave_rfi_autocorr_maxhold_acc_cnt_user_data_in/1 -> sim_out/1
  out_reg/1 -> sim_out_reg_sim_delay/1, assert_reg/1
  assert_reg/1 -> reint1/1
  reint1/1 -> io_delay/1

== system dsa2k_iwave_rfi/autocorr_maxhold/acc_len ==
  sim_1 : Inport
  convert1_1 : DataTypeConversion  OutDataTypeStr=fixdt('ufix32_En0')  LockScale=on
  convert2_1 : DataTypeConversion  OutDataTypeStr=fixdt('ufix32_En0')  ConvertRealWorld=Stored Integer (SI)  LockScale=on
  dsa2k_iwave_rfi_autocorr_maxhold_acc_len_user_data_out : xbsIndex_r4/Gateway In  gui_display_data_type=Fixed-point  arith_type=Unsigned  n_bits=32  bin_pt=0  preci_type=Single  exp_width=8  frac_width=24  rows=1  columns=1  quantization="Round  (unbiased: +/- Inf)"  overflow=Saturate  period=1  UseAsADC=off  ADCChannel='1'  interface=None  automatic_assignment=on  address_offset=hex2dec('00')  intf_name=''  intf_description=''  default_value=0  timing_constraint=None  locs_specified=off  LOCs={}  io_standard={}  inherit_from_input=off  hdl_port=on  dbl_ovrd=off  block_type=gatewayin
  gain_1 : Gain  OutDataTypeStr=fixdt('ufix32_En0')
  io_delay : xbsIndex_r4/Delay  rst=off  infoeditControl=Selection of Reset will increase slice count due to use of real FFs and instead of SRLs  en=off  latency=0  reg_retiming=on  dbl_ovrd=off  block_type=delay
  reint1 : xbsIndex_r4/Reinterpret  force_arith_type=on  arith_type=Unsigned  force_bin_pt=on  bin_pt=0  block_type=reinterpret
  slice_reg : xbsIndex_r4/Slice  nbits=32  boolean_output=off  mode=Lower Bit Location + Width  bit1=0  base1=MSB of Input  bit0=0  base0=LSB of Input  dbl_ovrd=off  block_type=slice
  in_reg : Outport  VectorParamsAs1DForOutWhenUnconnected=off
  wires:
  dsa2k_iwave_rfi_autocorr_maxhold_acc_len_user_data_out/1 -> io_delay/1
  sim_1/1 -> convert1_1/1
  convert1_1/1 -> convert2_1/1
  convert2_1/1 -> gain_1/1
  gain_1/1 -> dsa2k_iwave_rfi_autocorr_maxhold_acc_len_user_data_out/1
  io_delay/1 -> slice_reg/1
  slice_reg/1 -> reint1/1
  reint1/1 -> in_reg/1

== system dsa2k_iwave_rfi/autocorr_maxhold/block_info ==
  info : Subsystem  Tag=casper:info  mask(comment_block){info={"library":"rtr","block_type":"rtr:autocorr-maxhold","block_name":"dsa2k_iwave_rfi/autocorr_maxhold","rev_major":1,"rev_minor":0,"n_chan_serial_bits":11,"n_chan_parallel_bits":3,"n_input_serial_bits":0,"n_input":2}}
      mask help:
      | Any comment made using this block will be parsed by the toolflow and stored in the bitstream, accessible by software.
      | It's an unevaluated string, and some characters make Matlab unhappy, so the user must define/find a data transport format if that is the intended purpose.
      settings: MoveFcn=pos = get_param(gcb, 'Position'); height = pos(4)-pos(2); txt = get_param(gcb, 'info'); set_param(gcb,'MaskValueString',txt);
      mask Display:
      | pos = get_param(gcb, 'Position');
      | height = pos(4)-pos(2);
      | txt = get_param(gcb, 'info');
      | text(10,height/2,txt);

== system dsa2k_iwave_rfi/autocorr_maxhold/bus_expand ==
  bus_in : Inport
  reinterpret1 : xbsIndex_r4/Reinterpret  force_arith_type=on  arith_type=Unsigned  force_bin_pt=on  bin_pt=0  block_type=reinterpret
  reinterpret2 : xbsIndex_r4/Reinterpret  force_arith_type=on  arith_type=Unsigned  force_bin_pt=on  bin_pt=0  block_type=reinterpret
  slice1 : xbsIndex_r4/Slice  nbits=288  boolean_output=off  mode=Upper Bit Location + Width  bit1=-288  base1=MSB of Input  bit0=0  base0=LSB of Input  dbl_ovrd=off  block_type=slice
  slice2 : xbsIndex_r4/Slice  nbits=288  boolean_output=off  mode=Upper Bit Location + Width  bit1=0  base1=MSB of Input  bit0=0  base0=LSB of Input  dbl_ovrd=off  block_type=slice
  msb_out2 : Outport  VectorParamsAs1DForOutWhenUnconnected=off
  lsb_out1 : Outport  Port=2  VectorParamsAs1DForOutWhenUnconnected=off
  wires:
  bus_in/1 -> slice2/1, slice1/1
  slice2/1 -> reinterpret2/1
  reinterpret2/1 -> msb_out2/1
  slice1/1 -> reinterpret1/1
  reinterpret1/1 -> lsb_out1/1

== system dsa2k_iwave_rfi/autocorr_maxhold/trig ==
  sim_1 : Inport
  convert1_1 : DataTypeConversion  OutDataTypeStr=fixdt('ufix1_En0')  LockScale=on
  convert2_1 : DataTypeConversion  OutDataTypeStr=fixdt('ufix1_En0')  ConvertRealWorld=Stored Integer (SI)  LockScale=on
  dsa2k_iwave_rfi_autocorr_maxhold_trig_user_data_out : xbsIndex_r4/Gateway In  gui_display_data_type=Fixed-point  arith_type=Unsigned  n_bits=32  bin_pt=0  preci_type=Single  exp_width=8  frac_width=24  rows=1  columns=1  quantization="Round  (unbiased: +/- Inf)"  overflow=Saturate  period=1  UseAsADC=off  ADCChannel='1'  interface=None  automatic_assignment=on  address_offset=hex2dec('00')  intf_name=''  intf_description=''  default_value=0  timing_constraint=None  locs_specified=off  LOCs={}  io_standard={}  inherit_from_input=off  hdl_port=on  dbl_ovrd=off  block_type=gatewayin
  gain_1 : Gain  OutDataTypeStr=fixdt('ufix32_En0')
  io_delay : xbsIndex_r4/Delay  rst=off  infoeditControl=Selection of Reset will increase slice count due to use of real FFs and instead of SRLs  en=off  latency=0  reg_retiming=on  dbl_ovrd=off  block_type=delay
  slice_reg : xbsIndex_r4/Slice  nbits=1  boolean_output=on  mode=Lower Bit Location + Width  bit1=0  base1=MSB of Input  bit0=0  base0=LSB of Input  dbl_ovrd=off  block_type=slice
  in_reg : Outport  VectorParamsAs1DForOutWhenUnconnected=off
  wires:
  dsa2k_iwave_rfi_autocorr_maxhold_trig_user_data_out/1 -> io_delay/1
  sim_1/1 -> convert1_1/1
  convert1_1/1 -> convert2_1/1
  convert2_1/1 -> gain_1/1
  gain_1/1 -> dsa2k_iwave_rfi_autocorr_maxhold_trig_user_data_out/1
  io_delay/1 -> slice_reg/1
  slice_reg/1 -> in_reg/1

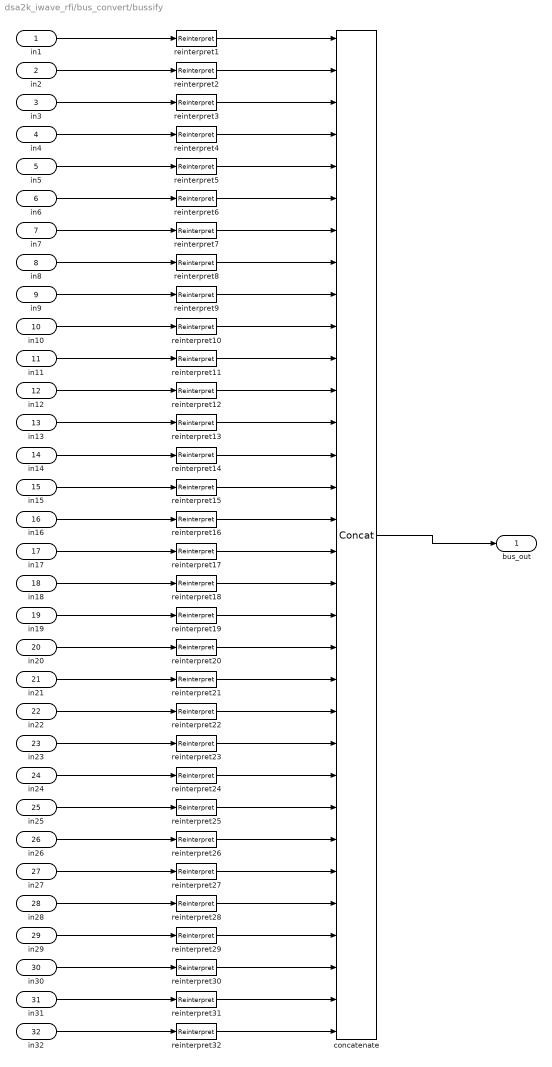
== system dsa2k_iwave_rfi/bus_convert/bussify ==
  in1 : Inport
  in2 : Inport  Port=2
  in3 : Inport  Port=3
  in4 : Inport  Port=4
  in5 : Inport  Port=5
  in6 : Inport  Port=6
  in7 : Inport  Port=7
  in8 : Inport  Port=8
  in9 : Inport  Port=9
  in10 : Inport  Port=10
  in11 : Inport  Port=11
  in12 : Inport  Port=12
  in13 : Inport  Port=13
  in14 : Inport  Port=14
  in15 : Inport  Port=15
  in16 : Inport  Port=16
  in17 : Inport  Port=17
  in18 : Inport  Port=18
  in19 : Inport  Port=19
  in20 : Inport  Port=20
  in21 : Inport  Port=21
  in22 : Inport  Port=22
  in23 : Inport  Port=23
  in24 : Inport  Port=24
  in25 : Inport  Port=25
  in26 : Inport  Port=26
  in27 : Inport  Port=27
  in28 : Inport  Port=28
  in29 : Inport  Port=29
  in30 : Inport  Port=30
  in31 : Inport  Port=31
  in32 : Inport  Port=32
  concatenate : xbsIndex_r4/Concat  num_inputs=32  dbl_ovrd=off  block_type=concat
  reinterpret{1..32} (32 alike) : xbsIndex_r4/Reinterpret  force_arith_type=on  arith_type=Unsigned  force_bin_pt=on  bin_pt=0  block_type=reinterpret
      reinterpret1 settings: infoedit="Changes signal type without altering the binary representation.   You can changed the signal between signed and unsigned, and relocate the binary point.<br><br>Hardware notes: In hardware this block costs nothing.<br><br>Example:  Suppose the input is 6 bits wide, signed, with 2 fractional bits, and the output is forced to unsigned with 0 fractional bits.  Then an input of -2.0 (1110.00 in binary 2's complement) becomes an output of 56 (111000 in binary)."
      reinterpret2 settings: infoedit="Changes signal type without altering the binary representation.   You can changed the signal between signed and unsigned, and relocate the binary point.<br><br>Hardware notes: In hardware this block costs nothing.<br><br>Example:  Suppose the input is 6 bits wide, signed, with 2 fractional bits, and the output is forced to unsigned with 0 fractional bits.  Then an input of -2.0 (1110.00 in binary 2's complement) becomes an output of 56 (111000 in binary)."
  bus_out : Outport  VectorParamsAs1DForOutWhenUnconnected=off
  wires:
  concatenate/1 -> bus_out/1
  in1/1 -> reinterpret1/1
  reinterpret1/1 -> concatenate/1
  in2/1 -> reinterpret2/1
  reinterpret2/1 -> concatenate/2
  in3/1 -> reinterpret3/1
  reinterpret3/1 -> concatenate/3
  in4/1 -> reinterpret4/1
  reinterpret4/1 -> concatenate/4
  in5/1 -> reinterpret5/1
  reinterpret5/1 -> concatenate/5
  in6/1 -> reinterpret6/1
  reinterpret6/1 -> concatenate/6
  in7/1 -> reinterpret7/1
  reinterpret7/1 -> concatenate/7
  in8/1 -> reinterpret8/1
  reinterpret8/1 -> concatenate/8
  in9/1 -> reinterpret9/1
  reinterpret9/1 -> concatenate/9
  in10/1 -> reinterpret10/1
  reinterpret10/1 -> concatenate/10
  in11/1 -> reinterpret11/1
  reinterpret11/1 -> concatenate/11
  in12/1 -> reinterpret12/1
  reinterpret12/1 -> concatenate/12
  in13/1 -> reinterpret13/1
  reinterpret13/1 -> concatenate/13
  in14/1 -> reinterpret14/1
  reinterpret14/1 -> concatenate/14
  in15/1 -> reinterpret15/1
  reinterpret15/1 -> concatenate/15
  in16/1 -> reinterpret16/1
  reinterpret16/1 -> concatenate/16
  in17/1 -> reinterpret17/1
  reinterpret17/1 -> concatenate/17
  in18/1 -> reinterpret18/1
  reinterpret18/1 -> concatenate/18
  in19/1 -> reinterpret19/1
  reinterpret19/1 -> concatenate/19
  in20/1 -> reinterpret20/1
  reinterpret20/1 -> concatenate/20
  in21/1 -> reinterpret21/1
  reinterpret21/1 -> concatenate/21
  in22/1 -> reinterpret22/1
  reinterpret22/1 -> concatenate/22
  in23/1 -> reinterpret23/1
  reinterpret23/1 -> concatenate/23
  in24/1 -> reinterpret24/1
  reinterpret24/1 -> concatenate/24
  in25/1 -> reinterpret25/1
  reinterpret25/1 -> concatenate/25
  in26/1 -> reinterpret26/1
  reinterpret26/1 -> concatenate/26
  in27/1 -> reinterpret27/1
  reinterpret27/1 -> concatenate/27
  in28/1 -> reinterpret28/1
  reinterpret28/1 -> concatenate/28
  in29/1 -> reinterpret29/1
  reinterpret29/1 -> concatenate/29
  in30/1 -> reinterpret30/1
  reinterpret30/1 -> concatenate/30
  in31/1 -> reinterpret31/1
  reinterpret31/1 -> concatenate/31
  in32/1 -> reinterpret32/1
  reinterpret32/1 -> concatenate/32
